simulink model "Filtro_de_emissao"  (R2013a)
settings: Solver=FixedStepDiscrete  StartTime=0.0  StopTime=10.0  RelTol=1e-3
settings Model: Creator=Élio  LastModifiedBy=Élio
settings OptimizationCC: InlineParams=on

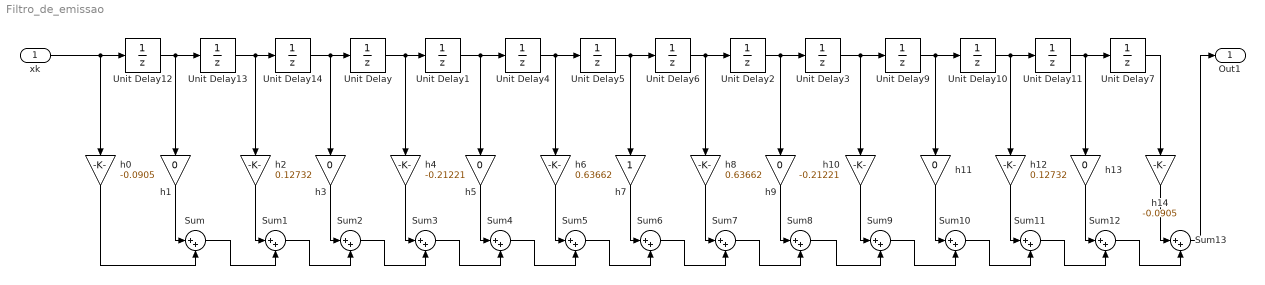
== system Filtro_de_emissao ==
  xk : Inport
  Sum{,1..13} (14 alike) : Sum  Inputs=|++
  Unit Delay{,1..7,9..14} (14 alike) : UnitDelay  SampleTime=-1
  h0 : Gain  Gain=-0.0905
  h{1,3,5,9,11,13} (6 alike) : Gain  Gain=0
  h10 : Gain  Gain=-0.21221
  h12 : Gain  Gain=0.12732
  h14 : Gain  Gain=-0.0905
  h2 : Gain  Gain=0.12732
  h4 : Gain  Gain=-0.21221
  h6 : Gain  Gain=0.63662
  h7 : Gain
  h8 : Gain  Gain=0.63662
  Out1 : Outport
  wires:
  Unit Delay12/1 -> Unit Delay13/1, h1/1
  Unit Delay13/1 -> Unit Delay14/1, h2/1
  Unit Delay14/1 -> Unit Delay/1, h3/1
  Unit Delay/1 -> Unit Delay1/1, h4/1
  Unit Delay1/1 -> Unit Delay4/1, h5/1
  Unit Delay4/1 -> Unit Delay5/1, h6/1
  Unit Delay5/1 -> Unit Delay6/1, h7/1
  Unit Delay6/1 -> Unit Delay2/1, h8/1
  Unit Delay2/1 -> Unit Delay3/1, h9/1
  Unit Delay3/1 -> Unit Delay9/1, h10/1
  Unit Delay9/1 -> Unit Delay10/1, h11/1
  Unit Delay10/1 -> Unit Delay11/1, h12/1
  Unit Delay11/1 -> Unit Delay7/1, h13/1
  Unit Delay7/1 -> h14/1
  h1/1 -> Sum/1
  h0/1 -> Sum/2
  xk/1 -> Unit Delay12/1, h0/1
  Sum/1 -> Sum1/2
  h2/1 -> Sum1/1
  h3/1 -> Sum2/1
  h4/1 -> Sum3/1
  h5/1 -> Sum4/1
  h6/1 -> Sum5/1
  h7/1 -> Sum6/1
  h8/1 -> Sum7/1
  h9/1 -> Sum8/1
  h10/1 -> Sum9/1
  h11/1 -> Sum10/1
  h12/1 -> Sum11/1
  h13/1 -> Sum12/1
  h14/1 -> Sum13/1
  Sum1/1 -> Sum2/2
  Sum2/1 -> Sum3/2
  Sum3/1 -> Sum4/2
  Sum4/1 -> Sum5/2
  Sum5/1 -> Sum6/2
  Sum6/1 -> Sum7/2
  Sum7/1 -> Sum8/2
  Sum8/1 -> Sum9/2
  Sum9/1 -> Sum10/2
  Sum10/1 -> Sum11/2
  Sum11/1 -> Sum12/2
  Sum12/1 -> Sum13/2
  Sum13/1 -> Out1/1
